simulink model "controllers"  (R2019b)
settings: Solver=VariableStepAuto  StartTime=0.0  StopTime=160  RelTol=1e-3
values from neighbouring files (symbols this model uses):
  Alat = [-0.1180 32.033 0 0 ... (first row only)    [model.m]
  Blat = [0 ... (first row only)    [model.m]
  Clat = [0.3048 0 0 0]    [model.m]
  Dlat = 0    [model.m]
undefined symbols (not defined in the file or in its folder): cf_den, cf_num, DEN, fl, Ki, Kp, NUM
libraries: simulink_extras x1
settings Model: Creator=Merc  LastModifiedBy=brian
settings SolverCC: ZeroCrossAlgorithm=Adaptive
settings DataIOCC: ReturnWorkspaceOutputs=off
settings DebuggingCC: IgnoredZcDiagnostic=none  ArithmeticOperatorsInVariantConditions=warning
settings SFSimCC: CustomCodeUndefinedFunction=UseInterfaceOnly

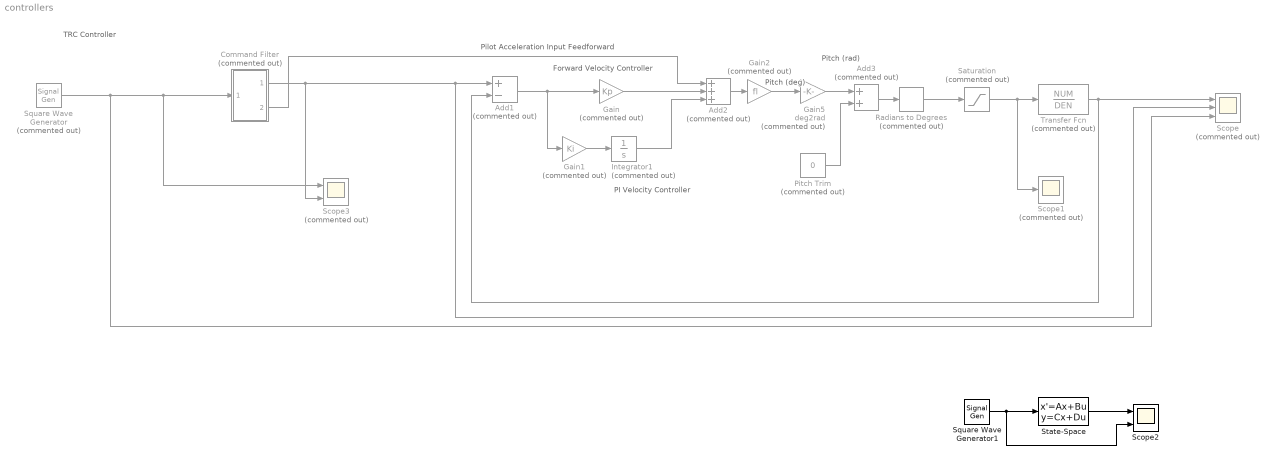
== system controllers ==
  note: TRC Controller
  note: Pitch (rad)
  note: Pitch (deg)
  note: Forward Velocity Controller
  note: PI Velocity Controller
  note: Pilot Acceleration Input Feedforward
  Add1 : Sum  Commented=on  Inputs=+-
  Add2 : Sum  Commented=on  Inputs=+++
  Add3 : Sum  Commented=on
  Command Filter : Subsystem  Commented=on
  Gain : Gain  Commented=on  Gain=Kp
  Gain1 : Gain  Commented=on  Gain=Ki
  Gain2 : Gain  Commented=on  Gain=fl
  Gain5 : Gain  Commented=on  Gain=deg2rad
  Integrator1 : Integrator  Commented=on
  Pitch Trim : Constant  Commented=on  Value=0
  Radians to Degrees : simulink_extras/Transformations/Radians to Degrees  Commented=on
  Saturation : Saturate  Commented=on  UpperLimit=400  LowerLimit=-400
  Scope : Scope  Commented=on  NumInputPorts=3
  Scope1 : Scope  Commented=on
  Scope2 : Scope  NumInputPorts=2
  Scope3 : Scope  Commented=on  NumInputPorts=2
  Square Wave Generator : SignalGenerator  Commented=on  WaveForm=square  Frequency=0.25  Units=rad/sec
  Square Wave Generator1 : SignalGenerator  WaveForm=square  Frequency=0.25  Units=rad/sec
  State-Space : StateSpace  A=Alat  B=Blat  C=Clat  D=Dlat  InitialCondition=0
  Transfer Fcn : TransferFcn  Commented=on  Numerator=NUM  Denominator=DEN
  wires:
  Add1/1 -> Gain1/1, Gain/1
  Gain/1 -> Add2/2
  Add2/1 -> Gain2/1
  Pitch Trim/1 -> Add3/2
  Transfer Fcn/1 -> Add1/2, Scope/1
  Gain5/1 -> Add3/1
  Gain2/1 -> Gain5/1
  Command Filter/1(Out1) -> Scope/2, Add1/1, Scope3/2
  Command Filter/2(Out2) -> Add2/1
  Add3/1 -> Radians to Degrees/1
  Square Wave Generator/1 -> Scope/3, Scope3/1, Command Filter/1(In1)
  Gain1/1 -> Integrator1/1
  Integrator1/1 -> Add2/3
  Radians to Degrees/1 -> Saturation/1
  Saturation/1 -> Scope1/1, Transfer Fcn/1
  State-Space/1 -> Scope2/1
  Square Wave Generator1/1 -> Scope2/2, State-Space/1

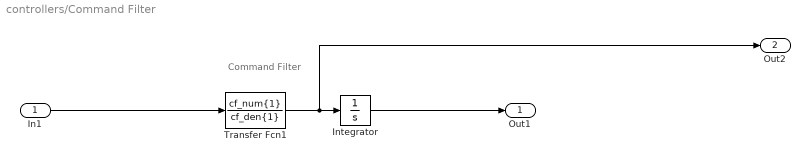
== system controllers/Command Filter ==
  note: Command Filter
  In1 : Inport
  Integrator : Integrator
  Transfer Fcn1 : TransferFcn  Numerator=cf_num{1}  Denominator=cf_den{1}
  Out1 : Outport  VectorParamsAs1DForOutWhenUnconnected=off
  Out2 : Outport  Port=2  VectorParamsAs1DForOutWhenUnconnected=off
  wires:
  Integrator/1 -> Out1/1
  In1/1 -> Transfer Fcn1/1
  Transfer Fcn1/1 -> Out2/1, Integrator/1
